simulink model "r2dbe_top"  (R2012b)
settings: Solver=VariableStepDiscrete  SolverMode=SingleTasking  StartTime=0.0  StopTime=10000  RelTol=1e-3
undefined symbols (not defined in the file or in its folder): r2dbe_vdif_lib, sfp, vdif
libraries: xbsIndex_r4 x2792, dspsigops x32, casper_library_delays x29, casper_library_sources x16, casper_library_misc x12, r2dbe_adc_lib x5, xps_library x4, simulink x2
(part 10 of 28)

== system r2dbe_top/r2dbe/tengbe_1/dest_ip ==
  sim_1 : Inport
  io_delay : xbsIndex_r4/Delay  rst=off  infoeditControl=Selection of Reset will increase slice count due to use of real FFs and instead of SRLs  en=off  latency=0  dbl_ovrd=off  reg_retiming=on  block_type=delay
  r2dbe_top_r2dbe_tengbe_1_dest_ip_user_data_out : xbsIndex_r4/Gateway In  gui_display_data_type=Fixed-point  arith_type=Unsigned  n_bits=32  bin_pt=0  preci_type=Single  exp_width=8  frac_width=24  quantization="Round  (unbiased: +/- Inf)"  overflow=Saturate  period=1  dbl_ovrd=off  timing_constraint=None  locs_specified=off  LOCs={}  UseAsADC=off  ADCChannel='1'  inherit_from_input=off  hdl_port=on  block_type=gatewayin
  reint1 : xbsIndex_r4/Reinterpret  force_arith_type=on  arith_type=Unsigned  force_bin_pt=on  bin_pt=0  block_type=reinterpret
  slice_ip : xbsIndex_r4/Slice  nbits=32  boolean_output=off  mode=Lower Bit Location + Width  bit1=0  base1=MSB of Input  bit0=0  base0=LSB of Input  dbl_ovrd=off  block_type=slice
  in_ip : Outport
  wires:
  r2dbe_top_r2dbe_tengbe_1_dest_ip_user_data_out/1 -> io_delay/1
  sim_1/1 -> r2dbe_top_r2dbe_tengbe_1_dest_ip_user_data_out/1
  io_delay/1 -> slice_ip/1
  slice_ip/1 -> reint1/1
  reint1/1 -> in_ip/1

== system r2dbe_top/r2dbe/tengbe_1/dest_port ==
  sim_1 : Inport
  io_delay : xbsIndex_r4/Delay  rst=off  infoeditControl=Selection of Reset will increase slice count due to use of real FFs and instead of SRLs  en=off  latency=0  dbl_ovrd=off  reg_retiming=on  block_type=delay
  r2dbe_top_r2dbe_tengbe_1_dest_port_user_data_out : xbsIndex_r4/Gateway In  gui_display_data_type=Fixed-point  arith_type=Unsigned  n_bits=32  bin_pt=0  preci_type=Single  exp_width=8  frac_width=24  quantization="Round  (unbiased: +/- Inf)"  overflow=Saturate  period=1  dbl_ovrd=off  timing_constraint=None  locs_specified=off  LOCs={}  UseAsADC=off  ADCChannel='1'  inherit_from_input=off  hdl_port=on  block_type=gatewayin
  reint1 : xbsIndex_r4/Reinterpret  force_arith_type=on  arith_type=Unsigned  force_bin_pt=on  bin_pt=0  block_type=reinterpret
  slice_port : xbsIndex_r4/Slice  nbits=16  boolean_output=off  mode=Lower Bit Location + Width  bit1=0  base1=MSB of Input  bit0=0  base0=LSB of Input  dbl_ovrd=off  block_type=slice
  in_port : Outport
  wires:
  r2dbe_top_r2dbe_tengbe_1_dest_port_user_data_out/1 -> io_delay/1
  sim_1/1 -> r2dbe_top_r2dbe_tengbe_1_dest_port_user_data_out/1
  io_delay/1 -> slice_port/1
  slice_port/1 -> reint1/1
  reint1/1 -> in_port/1

== system r2dbe_top/r2dbe/tengbe_1/rst ==
  sim_1 : Inport
  io_delay : xbsIndex_r4/Delay  rst=off  infoeditControl=Selection of Reset will increase slice count due to use of real FFs and instead of SRLs  en=off  latency=0  dbl_ovrd=off  reg_retiming=on  block_type=delay
  r2dbe_top_r2dbe_tengbe_1_rst_user_data_out : xbsIndex_r4/Gateway In  gui_display_data_type=Fixed-point  arith_type=Unsigned  n_bits=32  bin_pt=0  preci_type=Single  exp_width=8  frac_width=24  quantization="Round  (unbiased: +/- Inf)"  overflow=Saturate  period=1  dbl_ovrd=off  timing_constraint=None  locs_specified=off  LOCs={}  UseAsADC=off  ADCChannel='1'  inherit_from_input=off  hdl_port=on  block_type=gatewayin
  reint1 : xbsIndex_r4/Reinterpret  force_arith_type=on  arith_type=Unsigned  force_bin_pt=on  bin_pt=0  block_type=reinterpret
  slice_ip : xbsIndex_r4/Slice  nbits=32  boolean_output=off  mode=Lower Bit Location + Width  bit1=0  base1=MSB of Input  bit0=0  base0=LSB of Input  dbl_ovrd=off  block_type=slice
  in_ip : Outport
  wires:
  r2dbe_top_r2dbe_tengbe_1_rst_user_data_out/1 -> io_delay/1
  sim_1/1 -> r2dbe_top_r2dbe_tengbe_1_rst_user_data_out/1
  io_delay/1 -> slice_ip/1
  slice_ip/1 -> reint1/1
  reint1/1 -> in_ip/1

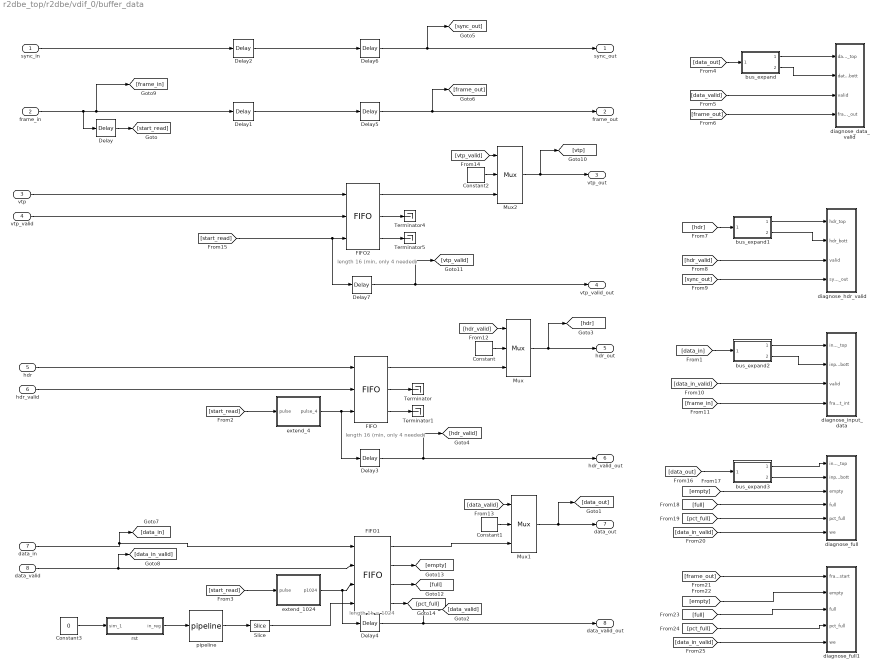
== system r2dbe_top/r2dbe/vdif_0/buffer_data ==
  note: length 1k = 1024
  note: length 16 (min, only 4 needed)
  note: length 16 (min, only 4 needed)
  sync_in : Inport
  frame_in : Inport  Port=2
  vtp : Inport  Port=3
  vtp_valid : Inport  Port=4
  hdr : Inport  Port=5
  hdr_valid : Inport  Port=6
  data_in : Inport  Port=7
  data_valid : Inport  Port=8
  Constant : xbsIndex_r4/Constant  const=0  gui_display_data_type=Fixed-point  arith_type=Unsigned  n_bits=64  bin_pt=0  preci_type=Single  exp_width=8  frac_width=24  explicit_period=on  period=1  equ=P=C  opselect=C  inp2=PCIN>>17  opr=+  inp1=P  carry=CIN  dbl_ovrd=off  block_type=constant
  Constant1 : xbsIndex_r4/Constant  const=0  gui_display_data_type=Fixed-point  arith_type=Unsigned  n_bits=64  bin_pt=0  preci_type=Single  exp_width=8  frac_width=24  explicit_period=on  period=1  equ=P=C  opselect=C  inp2=PCIN>>17  opr=+  inp1=P  carry=CIN  dbl_ovrd=off  block_type=constant
  Constant2 : xbsIndex_r4/Constant  const=0  gui_display_data_type=Fixed-point  arith_type=Unsigned  n_bits=64  bin_pt=0  preci_type=Single  exp_width=8  frac_width=24  explicit_period=on  period=1  equ=P=C  opselect=C  inp2=PCIN>>17  opr=+  inp1=P  carry=CIN  dbl_ovrd=off  block_type=constant
  Constant3 : Constant  Value=0
  Delay : xbsIndex_r4/Delay  rst=off  infoeditControl=Selection of Reset will increase slice count due to use of real FFs and instead of SRLs  en=off  latency=1024  dbl_ovrd=off  reg_retiming=off  block_type=delay
  Delay1 : xbsIndex_r4/Delay  rst=off  infoeditControl=Selection of Reset will increase slice count due to use of real FFs and instead of SRLs  en=off  latency=1024  dbl_ovrd=off  reg_retiming=off  block_type=delay
  Delay2 : xbsIndex_r4/Delay  rst=off  infoeditControl=Selection of Reset will increase slice count due to use of real FFs and instead of SRLs  en=off  latency=1024  dbl_ovrd=off  reg_retiming=off  block_type=delay
  Delay{3..7} (5 alike) : xbsIndex_r4/Delay  rst=off  infoeditControl=Selection of Reset will increase slice count due to use of real FFs and instead of SRLs  en=off  latency=1  dbl_ovrd=off  reg_retiming=off  block_type=delay
  FIFO : xbsIndex_r4/FIFO  mem_type=Block RAM  performance_options=Standard_FIFO  infoedit1=Available only for V4, V5, V6, V7, K7, A7 and Zynq devices.  embedded_registers=off  depth=16  percent_nbits=1  rst=off  en=off  use_dcount=off  use_percent_full_port=off  use_almost_empty=off  almost_empty_thresh=2  use_almost_full=off  almost_full_thresh=14  dbl_ovrd=off  explicit_period=off  block_type=fifo
  FIFO1 : xbsIndex_r4/FIFO  mem_type=Block RAM  performance_options=Standard_FIFO  infoedit1=Available only for V4, V5, V6, V7, K7, A7 and Zynq devices.  embedded_registers=off  depth=1K  percent_nbits=6  rst=on  en=off  use_dcount=off  use_percent_full_port=on  use_almost_empty=off  almost_empty_thresh=2  use_almost_full=off  almost_full_thresh=14  dbl_ovrd=off  explicit_period=off  block_type=fifo
  FIFO2 : xbsIndex_r4/FIFO  mem_type=Block RAM  performance_options=Standard_FIFO  infoedit1=Available only for V4, V5, V6, V7, K7, A7 and Zynq devices.  embedded_registers=off  depth=16  percent_nbits=1  rst=off  en=off  use_dcount=off  use_percent_full_port=off  use_almost_empty=off  almost_empty_thresh=2  use_almost_full=off  almost_full_thresh=14  dbl_ovrd=off  explicit_period=off  block_type=fifo
  Mux : xbsIndex_r4/Mux  inputs=2  en=off  latency=0  precision=Full  arith_type=Unsigned  n_bits=16  bin_pt=14  quantization=Truncate  overflow=Wrap  dbl_ovrd=off  block_type=mux
  Mux1 : xbsIndex_r4/Mux  inputs=2  en=off  latency=0  precision=Full  arith_type=Unsigned  n_bits=16  bin_pt=14  quantization=Truncate  overflow=Wrap  dbl_ovrd=off  block_type=mux
  Mux2 : xbsIndex_r4/Mux  inputs=2  en=off  latency=0  precision=Full  arith_type=Unsigned  n_bits=16  bin_pt=14  quantization=Truncate  overflow=Wrap  dbl_ovrd=off  block_type=mux
  Slice : xbsIndex_r4/Slice  nbits=1  boolean_output=on  mode=Lower Bit Location + Width  bit1=0  base1=LSB of Input  bit0=0  base0=LSB of Input  dbl_ovrd=off  block_type=slice
  Terminator{,1,4..5} (4 alike) : Terminator
  bus_expand : Subsystem  AncestorBlock=casper_library_flow_control/bus_expand  mask(bus_expand){mode=divisions of equal size, outputNum=2, outputWidth=32, outputBinaryPt=0, outputArithmeticType=0, show_format=off, outputToWorkspace=off, variablePrefix=out, outputToModelAsWell=on}
      mask prompts: outputNum "Number of outputs:"; outputWidth "Output width:"; outputBinaryPt "Output binary point position:"; outputArithmeticType "Output arithmetic type (ufix=0, fix=1, bool=2):"; show_format "Print format string?"; outputToWorkspace "Output to workspace?"; variablePrefix "Variable name prefix:"; outputToModelAsWell "Output to model as well?"
      mask help:
      | Expands a 'bus' made using a bus_create or Xilinx
      | concat block.
      | The input will be divided into the specified number
      | of outputs with the specified arithmetic types.
      | Divisions are made from most significant bit.
      mask init: same as r2dbe_top/r2dbe/delay_0/unbus
      settings: AttributesFormatString=2 outputs
      mask TypeOptions mode: divisions of equal size | divisions of arbitrary size
      mask Callback mode: bus_expand_callback();
      mask Callback outputWidth: bus_expand_callback();
      mask Callback outputToWorkspace: bus_expand_callback();
  bus_expand1 : Subsystem  AncestorBlock=casper_library_flow_control/bus_expand  mask(bus_expand){mode=divisions of equal size, outputNum=2, outputWidth=32, outputBinaryPt=0, outputArithmeticType=0, show_format=off, outputToWorkspace=off, variablePrefix=out, outputToModelAsWell=on}
      mask prompts: outputNum "Number of outputs:"; outputWidth "Output width:"; outputBinaryPt "Output binary point position:"; outputArithmeticType "Output arithmetic type (ufix=0, fix=1, bool=2):"; show_format "Print format string?"; outputToWorkspace "Output to workspace?"; variablePrefix "Variable name prefix:"; outputToModelAsWell "Output to model as well?"
      mask help:
      | Expands a 'bus' made using a bus_create or Xilinx
      | concat block.
      | The input will be divided into the specified number
      | of outputs with the specified arithmetic types.
      | Divisions are made from most significant bit.
      mask init: same as r2dbe_top/r2dbe/delay_0/unbus
      settings: AttributesFormatString=2 outputs
      mask TypeOptions mode: divisions of equal size | divisions of arbitrary size
      mask Callback mode: bus_expand_callback();
      mask Callback outputWidth: bus_expand_callback();
      mask Callback outputToWorkspace: bus_expand_callback();
  bus_expand2 : Subsystem  AncestorBlock=casper_library_flow_control/bus_expand  mask(bus_expand){mode=divisions of equal size, outputNum=2, outputWidth=32, outputBinaryPt=0, outputArithmeticType=0, show_format=off, outputToWorkspace=off, variablePrefix=out, outputToModelAsWell=on}
      mask prompts: outputNum "Number of outputs:"; outputWidth "Output width:"; outputBinaryPt "Output binary point position:"; outputArithmeticType "Output arithmetic type (ufix=0, fix=1, bool=2):"; show_format "Print format string?"; outputToWorkspace "Output to workspace?"; variablePrefix "Variable name prefix:"; outputToModelAsWell "Output to model as well?"
      mask help:
      | Expands a 'bus' made using a bus_create or Xilinx
      | concat block.
      | The input will be divided into the specified number
      | of outputs with the specified arithmetic types.
      | Divisions are made from most significant bit.
      mask init: same as r2dbe_top/r2dbe/delay_0/unbus
      settings: AttributesFormatString=2 outputs
      mask TypeOptions mode: divisions of equal size | divisions of arbitrary size
      mask Callback mode: bus_expand_callback();
      mask Callback outputWidth: bus_expand_callback();
      mask Callback outputToWorkspace: bus_expand_callback();
  bus_expand3 : Subsystem  AncestorBlock=casper_library_flow_control/bus_expand  mask(bus_expand){mode=divisions of equal size, outputNum=2, outputWidth=32, outputBinaryPt=0, outputArithmeticType=0, show_format=off, outputToWorkspace=off, variablePrefix=out, outputToModelAsWell=on}
      mask prompts: outputNum "Number of outputs:"; outputWidth "Output width:"; outputBinaryPt "Output binary point position:"; outputArithmeticType "Output arithmetic type (ufix=0, fix=1, bool=2):"; show_format "Print format string?"; outputToWorkspace "Output to workspace?"; variablePrefix "Variable name prefix:"; outputToModelAsWell "Output to model as well?"
      mask help:
      | Expands a 'bus' made using a bus_create or Xilinx
      | concat block.
      | The input will be divided into the specified number
      | of outputs with the specified arithmetic types.
      | Divisions are made from most significant bit.
      mask init: same as r2dbe_top/r2dbe/delay_0/unbus
      settings: AttributesFormatString=2 outputs
      mask TypeOptions mode: divisions of equal size | divisions of arbitrary size
      mask Callback mode: bus_expand_callback();
      mask Callback outputWidth: bus_expand_callback();
      mask Callback outputToWorkspace: bus_expand_callback();
  diagnose_data_valid : Subsystem
  diagnose_full : Subsystem
  diagnose_full1 : Subsystem
  diagnose_hdr_valid : Subsystem
  diagnose_input_data : Subsystem
  extend_1024 : Subsystem
  extend_4 : Subsystem
  pipeline : casper_library_delays/pipeline  latency=3
      settings: AttributesFormatString=Latency = %<latency>
  rst : Subsystem  Tag=xps:sw_reg  AncestorBlock=xps_library/software register  mask(swreg){mode=one value, io_dir=From Processor, io_delay=0, sample_period=1, names=reg, bitwidths=32, arith_types=0, bin_pts=0, sim_port=on, show_format=off}
      mask prompts: io_dir "I/O direction"; io_delay "I/O delay"; sample_period "Sample period"; names "Name:"; bitwidths "Bitwidth:"; arith_types "Type (ufix=0, fix=1, bool=2):"; bin_pts "Binary pt:"; sim_port "Provide sim input/output?"; show_format "Print format string?"
      mask init:
      | swreg_init(gcb)
      settings: AttributesFormatString=1input
      mask TypeOptions mode: one value | fields of equal size | fields of arbitrary size
      mask Callback mode: swreg_cb(gcb);
      mask TypeOptions io_dir: To Processor | From Processor
      mask Callback io_dir:
      | mask_enables = get_param(gcb, 'MaskEnables');
      | mask_names = get_param(gcb, 'MaskNames');
      | if strcmp(get_param(gcb, 'io_dir'), 'To Processor'),
      |     mask_enables{ismember(mask_names, 'sample_period')} = 'off';
      | else
      |     mask_enables{ismember(mask_names, 'sample_period')} = 'on';
      | end
      | set_param(gcb, 'MaskEnables', mask_enables);
      mask Callback bitwidths:
      | swreg_maskcheck(gcb);
      | % blk = gcb;
      | % mode = get_param(blk, 'mode');
      | % current_widths = eval(get_param(blk, 'bitwidths'));
      | % if (strcmp(mode, 'one value') || strcmp(mode, 'fields of equal size')) && (length(current_widths) > 1),
      | %     error('Only one width may be specified for this mode.');
      | % elseif strcmp(mode, 'fields of arbitrary size')
      | %     current_names = textscan(strtrim(strrep(strrep(get_param(blk, 'names'), ']', ''), '[', '')), '%s');
      | %     current_names = current_names{1};
      | %     numios = length(current_names);
      | %     if length(current_widths) ~= numios,
      | %         error('%d field names specified, but %d widths?', numios, length(current_widths));
      | %     end
      | % end
      | % total_width = 0;
      | % for ctr = 1 : length(current_widths),
      | %     total_width = total_width + current_widths(ctr);
      | % end
      | % if total_width > 32,
      | %     error('Total width must be 32 or less, set to %d.', total_width);
      | % end
      mask Callback arith_types:
      | [numios, ~, ~, ~, current_types] = swreg_maskcheck(gcb);
      | % blk = gcb;
      | % mode = get_param(blk, 'mode');
      | % current_types = eval(get_param(blk, 'arith_types'));
      | % numios = length(current_types);
      | % if (strcmp(mode, 'one value') || strcmp(mode, 'fields of equal size')) && (length(current_types) > 1),
      | %     error('Only one type may be specified for this mode.');
      | % elseif strcmp(mode, 'fields of arbitrary size')
      | %     current_names = textscan(strtrim(strrep(strrep(get_param(blk, 'names'), ']', ''), '[', '')), '%s');
      | %     current_names = current_names{1};
      | %     numios = length(current_names);
      | %     if length(current_types) ~= numios,
      | %         error('%d field names specified, but %d types?', numios, length(current_types));
      | %     end
      | % end
      | problem = 0;
      | for ctr = 1 : numios,
      |     t = current_types(ctr);
      |     if (t < 0) || (t > 2),
      |         problem = t;
      |         ctr = numios + 1;
      |     end
      | end
      | if problem ~= 0,
      |     error('Type cannot be %i, must be 0, 1 or 2.', problem);
      | end
      mask Callback bin_pts:
      | swreg_maskcheck(gcb);
      | % blk = gcb;
      | % mode = get_param(blk, 'mode');
      | % current_bins = eval(get_param(blk, 'bin_pts'));
      | % if (strcmp(mode, 'one value') || strcmp(mode, 'fields of equal size')) && (length(current_bins) > 1),
      | %     error('Only one binary pt may be specified for this mode.');
      | % elseif strcmp(mode, 'fields of arbitrary size')
      | %     current_names = textscan(strtrim(strrep(strrep(get_param(blk, 'names'), ']', ''), '[', '')), '%s');
      | %     current_names = current_names{1};
      | %     numios = length(current_names);
      | %     if length(current_bins) ~= numios,
      | %         error('%d field names specified, but %d binary pts?', numios, length(current_bins));
      | %     end
      | % end
  sync_out : Outport
  frame_out : Outport  Port=2
  vtp_out : Outport  Port=3
  vtp_valid_out : Outport  Port=4
  hdr_out : Outport  Port=5
  hdr_valid_out : Outport  Port=6
  data_out : Outport  Port=7
  data_valid_out : Outport  Port=8
  wires:
  sync_in/1 -> Delay2/1
  Delay/1 -> [start_read]
  hdr/1 -> FIFO/1
  hdr_valid/1 -> FIFO/2
  [start_read] -> extend_4/1(pulse)
  extend_4/1(pulse_4) -> Delay3/1, FIFO/3
  FIFO/1 -> Mux/3
  data_in/1 -> [data_in], FIFO1/1
  data_valid/1 -> [data_in_valid], FIFO1/2
  [start_read] -> extend_1024/1(pulse)
  extend_1024/1(p1024) -> Delay4/1, FIFO1/3
  FIFO1/1 -> Mux1/3
  FIFO/2 -> Terminator/1
  FIFO/3 -> Terminator1/1
  FIFO1/2 -> [empty]
  FIFO1/3 -> [full]
  bus_expand/2(lsb_out1) -> diagnose_data_valid/2(data_bott)
  bus_expand/1(msb_out2) -> diagnose_data_valid/1(data_top)
  [data_valid] -> diagnose_data_valid/3(valid)
  [frame_out] -> diagnose_data_valid/4(frame_start_out)
  [data_out] -> bus_expand/1(bus_in)
  frame_in/1 -> Delay/1, [frame_in], Delay1/1
  bus_expand1/2(lsb_out1) -> diagnose_hdr_valid/2(hdr_bott)
  bus_expand1/1(msb_out2) -> diagnose_hdr_valid/1(hdr_top)
  [hdr_valid] -> diagnose_hdr_valid/3(valid)
  [sync_out] -> diagnose_hdr_valid/4(sync_out)
  [hdr] -> bus_expand1/1(bus_in)
  Delay1/1 -> Delay5/1
  Delay2/1 -> Delay6/1
  bus_expand2/2(lsb_out1) -> diagnose_input_data/2(input_data_bott)
  bus_expand2/1(msb_out2) -> diagnose_input_data/1(input_data_top)
  [data_in_valid] -> diagnose_input_data/3(valid)
  [frame_in] -> diagnose_input_data/4(frame_start_int)
  [data_in] -> bus_expand2/1(bus_in)
  Delay3/1 -> hdr_valid_out/1, [hdr_valid]
  Delay4/1 -> data_valid_out/1, [data_valid]
  Delay5/1 -> frame_out/1, [frame_out]
  Delay6/1 -> [sync_out], sync_out/1
  Constant/1 -> Mux/2
  Mux/1 -> hdr_out/1, [hdr]
  [hdr_valid] -> Mux/1
  Constant1/1 -> Mux1/2
  [data_valid] -> Mux1/1
  Mux1/1 -> data_out/1, [data_out]
  vtp/1 -> FIFO2/1
  vtp_valid/1 -> FIFO2/2
  [start_read] -> FIFO2/3, Delay7/1
  FIFO2/1 -> Mux2/3
  FIFO2/2 -> Terminator4/1
  FIFO2/3 -> Terminator5/1
  Delay7/1 -> vtp_valid_out/1, [vtp_valid]
  Constant2/1 -> Mux2/2
  Mux2/1 -> vtp_out/1, [vtp]
  [vtp_valid] -> Mux2/1
  bus_expand3/2(lsb_out1) -> diagnose_full/2(input_data_bott)
  bus_expand3/1(msb_out2) -> diagnose_full/1(input_data_top)
  [empty] -> diagnose_full/3(empty)
  [full] -> diagnose_full/4(full)
  [data_out] -> bus_expand3/1(bus_in)
  [pct_full] -> diagnose_full/5(pct_full)
  [data_in_valid] -> diagnose_full/6(we)
  FIFO1/4 -> [pct_full]
  [empty] -> diagnose_full1/2(empty)
  [full] -> diagnose_full1/3(full)
  [pct_full] -> diagnose_full1/4(pct_full)
  [data_in_valid] -> diagnose_full1/5(we)
  [frame_out] -> diagnose_full1/1(frame_start)
  rst/1(in_reg) -> pipeline/1
  pipeline/1 -> Slice/1
  Constant3/1 -> rst/1(sim_1)
  Slice/1 -> FIFO1/4

== system r2dbe_top/r2dbe/vdif_0/delay_data ==
  sync_in : Inport
  frame_in : Inport  Port=2
  vtp : Inport  Port=3
  vtp_valid : Inport  Port=4
  hdr : Inport  Port=5
  hdr_valid : Inport  Port=6
  data : Inport  Port=7
  data_valid : Inport  Port=8
  Delay : xbsIndex_r4/Delay  rst=off  infoeditControl=Selection of Reset will increase slice count due to use of real FFs and instead of SRLs  en=off  latency=4  dbl_ovrd=off  reg_retiming=off  block_type=delay
  Delay1 : xbsIndex_r4/Delay  rst=off  infoeditControl=Selection of Reset will increase slice count due to use of real FFs and instead of SRLs  en=off  latency=4  dbl_ovrd=off  reg_retiming=off  block_type=delay
  Delay{2..5} (4 alike) : xbsIndex_r4/Delay  rst=off  infoeditControl=Selection of Reset will increase slice count due to use of real FFs and instead of SRLs  en=off  latency=1  dbl_ovrd=off  reg_retiming=off  block_type=delay
  bus_expand : Subsystem  AncestorBlock=casper_library_flow_control/bus_expand  mask(bus_expand){mode=divisions of equal size, outputNum=2, outputWidth=32, outputBinaryPt=0, outputArithmeticType=0, show_format=off, outputToWorkspace=off, variablePrefix=out, outputToModelAsWell=on}
      mask prompts: outputNum "Number of outputs:"; outputWidth "Output width:"; outputBinaryPt "Output binary point position:"; outputArithmeticType "Output arithmetic type (ufix=0, fix=1, bool=2):"; show_format "Print format string?"; outputToWorkspace "Output to workspace?"; variablePrefix "Variable name prefix:"; outputToModelAsWell "Output to model as well?"
      mask help:
      | Expands a 'bus' made using a bus_create or Xilinx
      | concat block.
      | The input will be divided into the specified number
      | of outputs with the specified arithmetic types.
      | Divisions are made from most significant bit.
      mask init: same as r2dbe_top/r2dbe/delay_0/unbus
      settings: AttributesFormatString=2 outputs
      mask TypeOptions mode: divisions of equal size | divisions of arbitrary size
      mask Callback mode: bus_expand_callback();
      mask Callback outputWidth: bus_expand_callback();
      mask Callback outputToWorkspace: bus_expand_callback();
  bus_expand1 : Subsystem  AncestorBlock=casper_library_flow_control/bus_expand  mask(bus_expand){mode=divisions of equal size, outputNum=2, outputWidth=32, outputBinaryPt=0, outputArithmeticType=0, show_format=off, outputToWorkspace=off, variablePrefix=out, outputToModelAsWell=on}
      mask prompts: outputNum "Number of outputs:"; outputWidth "Output width:"; outputBinaryPt "Output binary point position:"; outputArithmeticType "Output arithmetic type (ufix=0, fix=1, bool=2):"; show_format "Print format string?"; outputToWorkspace "Output to workspace?"; variablePrefix "Variable name prefix:"; outputToModelAsWell "Output to model as well?"
      mask help:
      | Expands a 'bus' made using a bus_create or Xilinx
      | concat block.
      | The input will be divided into the specified number
      | of outputs with the specified arithmetic types.
      | Divisions are made from most significant bit.
      mask init: same as r2dbe_top/r2dbe/delay_0/unbus
      settings: AttributesFormatString=2 outputs
      mask TypeOptions mode: divisions of equal size | divisions of arbitrary size
      mask Callback mode: bus_expand_callback();
      mask Callback outputWidth: bus_expand_callback();
      mask Callback outputToWorkspace: bus_expand_callback();
  diagnose_data_valid : Subsystem
  diagnose_data_valid1 : Subsystem
  sync_out : Outport
  frame_out : Outport  Port=2
  vtp_out : Outport  Port=3
  vtp_valid_out : Outport  Port=4
  hdr_out : Outport  Port=5
  hdr_out_valid : Outport  Port=6
  data_out : Outport  Port=7
  data_out_valid : Outport  Port=8
  wires:
  [data_out] -> bus_expand/1(bus_in)
  bus_expand/1(msb_out2) -> diagnose_data_valid/1(data_top)
  bus_expand/2(lsb_out1) -> diagnose_data_valid/2(data_bott)
  sync_in/1 -> [sync_out], sync_out/1
  frame_in/1 -> [frame_out], frame_out/1
  hdr/1 -> Delay3/1
  hdr_valid/1 -> Delay2/1
  data/1 -> Delay4/1
  Delay/1 -> [data_out], data_out/1
  data_valid/1 -> Delay5/1
  Delay1/1 -> [data_valid], data_out_valid/1
  [hdr] -> bus_expand1/1(bus_in)
  bus_expand1/1(msb_out2) -> diagnose_data_valid/4(hdr_top)
  bus_expand1/2(lsb_out1) -> diagnose_data_valid/5(hdr_bott)
  [data_valid] -> diagnose_data_valid/3(data_valid)
  [hdr_valid] -> diagnose_data_valid/6(hdr_valid)
  [sync_out] -> diagnose_data_valid1/1(sync)
  [frame_out] -> diagnose_data_valid1/2(frame)
  [data_valid] -> diagnose_data_valid1/3(data_valid)
  [hdr_valid] -> diagnose_data_valid1/4(hdr_valid)
  vtp/1 -> vtp_out/1, [vtp]
  vtp_valid/1 -> vtp_valid_out/1, [vtp_valid]
  Delay2/1 -> [hdr_valid], hdr_out_valid/1
  Delay3/1 -> [hdr], hdr_out/1
  Delay4/1 -> Delay/1
  Delay5/1 -> Delay1/1

== system r2dbe_top/r2dbe/vdif_0/enable ==
  sim_1 : Inport
  io_delay : xbsIndex_r4/Delay  rst=off  infoeditControl=Selection of Reset will increase slice count due to use of real FFs and instead of SRLs  en=off  latency=0  dbl_ovrd=off  reg_retiming=on  block_type=delay
  r2dbe_top_r2dbe_vdif_0_enable_user_data_out : xbsIndex_r4/Gateway In  gui_display_data_type=Fixed-point  arith_type=Unsigned  n_bits=32  bin_pt=0  preci_type=Single  exp_width=8  frac_width=24  quantization="Round  (unbiased: +/- Inf)"  overflow=Saturate  period=1  dbl_ovrd=off  timing_constraint=None  locs_specified=off  LOCs={}  UseAsADC=off  ADCChannel='1'  inherit_from_input=off  hdl_port=on  block_type=gatewayin
  reint1 : xbsIndex_r4/Reinterpret  force_arith_type=on  arith_type=Unsigned  force_bin_pt=on  bin_pt=0  block_type=reinterpret
  slice_reg : xbsIndex_r4/Slice  nbits=32  boolean_output=off  mode=Lower Bit Location + Width  bit1=0  base1=MSB of Input  bit0=0  base0=LSB of Input  dbl_ovrd=off  block_type=slice
  in_reg : Outport
  wires:
  r2dbe_top_r2dbe_vdif_0_enable_user_data_out/1 -> io_delay/1
  sim_1/1 -> r2dbe_top_r2dbe_vdif_0_enable_user_data_out/1
  io_delay/1 -> slice_reg/1
  slice_reg/1 -> reint1/1
  reint1/1 -> in_reg/1

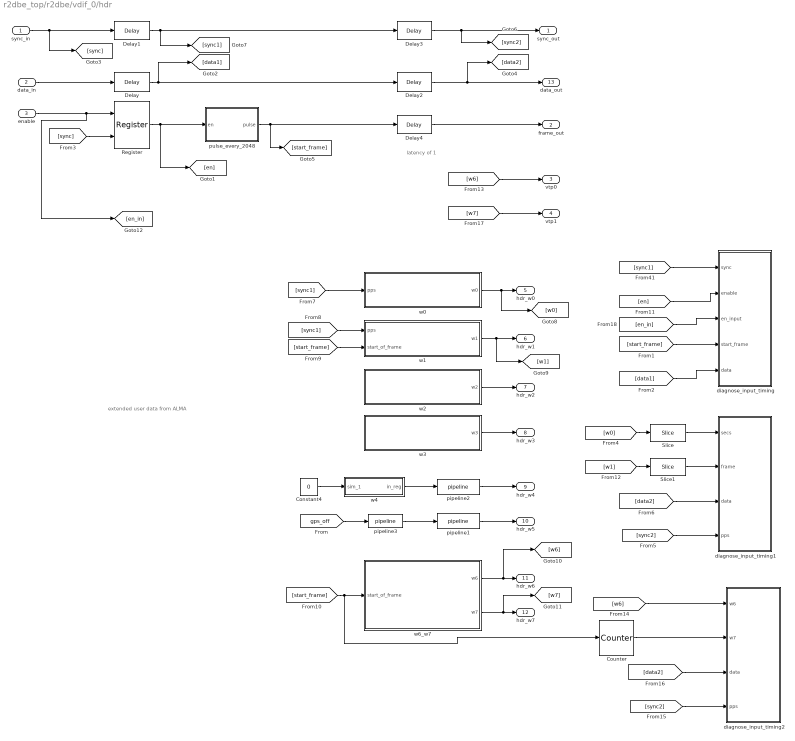
== system r2dbe_top/r2dbe/vdif_0/hdr ==
  note: latency of 1
  note: extended user data
      | from ALMA
  sync_in : Inport
  data_in : Inport  Port=2
  enable : Inport  Port=3
  Constant4 : Constant  Value=0
  Counter : xbsIndex_r4/Counter  cnt_type=Free Running  cnt_to=Inf  operation=Up  start_count=2^32-1  cnt_by_val=1  arith_type=Unsigned  n_bits=32  bin_pt=0  load_pin=off  rst=off  en=on  explicit_period=on  period=1  dbl_ovrd=off  use_behavioral_HDL=off  implementation=Fabric  block_type=counter
  Delay{,1..4} (5 alike) : xbsIndex_r4/Delay  rst=off  infoeditControl=Selection of Reset will increase slice count due to use of real FFs and instead of SRLs  en=off  latency=1  dbl_ovrd=off  reg_retiming=off  block_type=delay
  Register : xbsIndex_r4/Register  init=0  rst=off  en=on  dbl_ovrd=off  block_type=register
  Slice : xbsIndex_r4/Slice  nbits=30  boolean_output=off  mode=Lower Bit Location + Width  bit1=0  base1=MSB of Input  bit0=0  base0=LSB of Input  dbl_ovrd=off  block_type=slice
  Slice1 : xbsIndex_r4/Slice  nbits=24  boolean_output=off  mode=Lower Bit Location + Width  bit1=0  base1=MSB of Input  bit0=0  base0=LSB of Input  dbl_ovrd=off  block_type=slice
  diagnose_input_timing : Subsystem
  diagnose_input_timing1 : Subsystem
  diagnose_input_timing2 : Subsystem
  pipeline1 : casper_library_delays/pipeline  latency=1
      settings: AttributesFormatString=Latency = %<latency>
  pipeline2 : casper_library_delays/pipeline  latency=1
      settings: AttributesFormatString=Latency = %<latency>
  pipeline3 : casper_library_delays/pipeline  latency=3
      settings: AttributesFormatString=Latency = %<latency>
  pulse_every_2048 : Subsystem  mask{per=2048}
      mask prompts: per "period"
      mask help: Creates a pulse duration 1 with period from 2 to <large number>. Pulse begins with enable signal, no latency.
  w0 : Subsystem
  w1 : Subsystem
  w2 : Subsystem
  w3 : Subsystem
  w4 : Subsystem  Tag=xps:sw_reg  AncestorBlock=xps_library/software register  mask(swreg){mode=one value, io_dir=From Processor, io_delay=0, sample_period=1, names=reg, bitwidths=32, arith_types=0, bin_pts=0, sim_port=on, show_format=off}
      mask prompts: io_dir "I/O direction"; io_delay "I/O delay"; sample_period "Sample period"; names "Name:"; bitwidths "Bitwidth:"; arith_types "Type (ufix=0, fix=1, bool=2):"; bin_pts "Binary pt:"; sim_port "Provide sim input/output?"; show_format "Print format string?"
      mask init:
      | swreg_init(gcb)
      settings: AttributesFormatString=1input
      mask TypeOptions mode: one value | fields of equal size | fields of arbitrary size
      mask Callback mode: swreg_cb(gcb);
      mask TypeOptions io_dir: To Processor | From Processor
      mask Callback io_dir:
      | mask_enables = get_param(gcb, 'MaskEnables');
      | mask_names = get_param(gcb, 'MaskNames');
      | if strcmp(get_param(gcb, 'io_dir'), 'To Processor'),
      |     mask_enables{ismember(mask_names, 'sample_period')} = 'off';
      | else
      |     mask_enables{ismember(mask_names, 'sample_period')} = 'on';
      | end
      | set_param(gcb, 'MaskEnables', mask_enables);
      mask Callback bitwidths:
      | swreg_maskcheck(gcb);
      | % blk = gcb;
      | % mode = get_param(blk, 'mode');
      | % current_widths = eval(get_param(blk, 'bitwidths'));
      | % if (strcmp(mode, 'one value') || strcmp(mode, 'fields of equal size')) && (length(current_widths) > 1),
      | %     error('Only one width may be specified for this mode.');
      | % elseif strcmp(mode, 'fields of arbitrary size')
      | %     current_names = textscan(strtrim(strrep(strrep(get_param(blk, 'names'), ']', ''), '[', '')), '%s');
      | %     current_names = current_names{1};
      | %     numios = length(current_names);
      | %     if length(current_widths) ~= numios,
      | %         error('%d field names specified, but %d widths?', numios, length(current_widths));
      | %     end
      | % end
      | % total_width = 0;
      | % for ctr = 1 : length(current_widths),
      | %     total_width = total_width + current_widths(ctr);
      | % end
      | % if total_width > 32,
      | %     error('Total width must be 32 or less, set to %d.', total_width);
      | % end
      mask Callback arith_types:
      | [numios, ~, ~, ~, current_types] = swreg_maskcheck(gcb);
      | % blk = gcb;
      | % mode = get_param(blk, 'mode');
      | % current_types = eval(get_param(blk, 'arith_types'));
      | % numios = length(current_types);
      | % if (strcmp(mode, 'one value') || strcmp(mode, 'fields of equal size')) && (length(current_types) > 1),
      | %     error('Only one type may be specified for this mode.');
      | % elseif strcmp(mode, 'fields of arbitrary size')
      | %     current_names = textscan(strtrim(strrep(strrep(get_param(blk, 'names'), ']', ''), '[', '')), '%s');
      | %     current_names = current_names{1};
      | %     numios = length(current_names);
      | %     if length(current_types) ~= numios,
      | %         error('%d field names specified, but %d types?', numios, length(current_types));
      | %     end
      | % end
      | problem = 0;
      | for ctr = 1 : numios,
      |     t = current_types(ctr);
      |     if (t < 0) || (t > 2),
      |         problem = t;
      |         ctr = numios + 1;
      |     end
      | end
      | if problem ~= 0,
      |     error('Type cannot be %i, must be 0, 1 or 2.', problem);
      | end
      mask Callback bin_pts:
      | swreg_maskcheck(gcb);
      | % blk = gcb;
      | % mode = get_param(blk, 'mode');
      | % current_bins = eval(get_param(blk, 'bin_pts'));
      | % if (strcmp(mode, 'one value') || strcmp(mode, 'fields of equal size')) && (length(current_bins) > 1),
      | %     error('Only one binary pt may be specified for this mode.');
      | % elseif strcmp(mode, 'fields of arbitrary size')
      | %     current_names = textscan(strtrim(strrep(strrep(get_param(blk, 'names'), ']', ''), '[', '')), '%s');
      | %     current_names = current_names{1};
      | %     numios = length(current_names);
      | %     if length(current_bins) ~= numios,
      | %         error('%d field names specified, but %d binary pts?', numios, length(current_bins));
      | %     end
      | % end
  w6_w7 : Subsystem
  sync_out : Outport
  frame_out : Outport  Port=2
  vtp0 : Outport  Port=3
  vtp1 : Outport  Port=4
  hdr_w0 : Outport  Port=5
  hdr_w1 : Outport  Port=6
  hdr_w2 : Outport  Port=7
  hdr_w3 : Outport  Port=8
  hdr_w4 : Outport  Port=9
  hdr_w5 : Outport  Port=10
  hdr_w6 : Outport  Port=11
  hdr_w7 : Outport  Port=12
  data_out : Outport  Port=13
  wires:
  [gps_off] -> pipeline3/1
  w4/1(in_reg) -> pipeline2/1
  Constant4/1 -> w4/1(sim_1)
  [en] -> diagnose_input_timing/2(enable)
  [sync1] -> diagnose_input_timing/1(sync)
  [start_frame] -> w1/2(start_of_frame)
  [sync1] -> w1/1(pps)
  [sync1] -> w0/1(pps)
  sync_in/1 -> [sync], Delay1/1
  data_in/1 -> Delay/1
  w0/1(w0) -> hdr_w0/1, [w0]
  w1/1(w1) -> hdr_w1/1, [w1]
  w2/1(w2) -> hdr_w2/1
  w3/1(w3) -> hdr_w3/1
  pipeline2/1 -> hdr_w4/1
  pipeline1/1 -> hdr_w5/1
  w6_w7/1(w6) -> hdr_w6/1, [w6]
  w6_w7/2(w7) -> hdr_w7/1, [w7]
  [start_frame] -> Counter/1, w6_w7/1(start_of_frame)
  pulse_every_2048/1(pulse) -> Delay4/1, [start_frame]
  enable/1 -> [en_in], Register/1
  [sync] -> Register/2
  Register/1 -> [en], pulse_every_2048/1(en)
  Delay/1 -> [data1], Delay2/1
  Delay1/1 -> Delay3/1, [sync1]
  Slice1/1 -> diagnose_input_timing1/2(frame)
  Slice/1 -> diagnose_input_timing1/1(secs)
  [data2] -> diagnose_input_timing1/3(data)
  [sync2] -> diagnose_input_timing1/4(pps)
  Delay2/1 -> data_out/1, [data2]
  Delay3/1 -> [sync2], sync_out/1
  [w0] -> Slice/1
  [w1] -> Slice1/1
  Delay4/1 -> frame_out/1
  Counter/1 -> diagnose_input_timing2/2(w7)
  [w6] -> diagnose_input_timing2/1(w6)
  [data2] -> diagnose_input_timing2/3(data)
  [sync2] -> diagnose_input_timing2/4(pps)
  [w6] -> vtp0/1
  [w7] -> vtp1/1
  [en_in] -> diagnose_input_timing/3(en_input)
  [start_frame] -> diagnose_input_timing/4(start_frame)
  [data1] -> diagnose_input_timing/5(data)
  pipeline3/1 -> pipeline1/1

== system r2dbe_top/r2dbe/vdif_0/little_end ==
  sim_1 : Inport
  io_delay : xbsIndex_r4/Delay  rst=off  infoeditControl=Selection of Reset will increase slice count due to use of real FFs and instead of SRLs  en=off  latency=0  dbl_ovrd=off  reg_retiming=on  block_type=delay
  r2dbe_top_r2dbe_vdif_0_little_end_user_data_out : xbsIndex_r4/Gateway In  gui_display_data_type=Fixed-point  arith_type=Unsigned  n_bits=32  bin_pt=0  preci_type=Single  exp_width=8  frac_width=24  quantization="Round  (unbiased: +/- Inf)"  overflow=Saturate  period=1  dbl_ovrd=off  timing_constraint=None  locs_specified=off  LOCs={}  UseAsADC=off  ADCChannel='1'  inherit_from_input=off  hdl_port=on  block_type=gatewayin
  reint1 : xbsIndex_r4/Reinterpret  force_arith_type=on  arith_type=Unsigned  force_bin_pt=on  bin_pt=0  block_type=reinterpret
  slice_reg : xbsIndex_r4/Slice  nbits=32  boolean_output=off  mode=Lower Bit Location + Width  bit1=0  base1=MSB of Input  bit0=0  base0=LSB of Input  dbl_ovrd=off  block_type=slice
  in_reg : Outport
  wires:
  r2dbe_top_r2dbe_vdif_0_little_end_user_data_out/1 -> io_delay/1
  sim_1/1 -> r2dbe_top_r2dbe_vdif_0_little_end_user_data_out/1
  io_delay/1 -> slice_reg/1
  slice_reg/1 -> reint1/1
  reint1/1 -> in_reg/1

== system r2dbe_top/r2dbe/vdif_0/mk_64_from_32 ==
  sync_in : Inport
  frame_start : Inport  Port=2
  vtp : Inport  Port=3
  vtp_valid : Inport  Port=4
  hdr : Inport  Port=5
  hdr_valid : Inport  Port=6
  data_in : Inport  Port=7
  data_valid : Inport  Port=8
  Delay{,1..4} (5 alike) : xbsIndex_r4/Delay  rst=off  infoeditControl=Selection of Reset will increase slice count due to use of real FFs and instead of SRLs  en=off  latency=2  dbl_ovrd=off  reg_retiming=off  block_type=delay
  Logical : xbsIndex_r4/Logical  logical_function=AND  inputs=2  en=off  latency=0  precision=Full  arith_type=Unsigned  n_bits=16  bin_pt=0  align_bp=on  dbl_ovrd=off  block_type=logical
  Logical1 : xbsIndex_r4/Logical  logical_function=AND  inputs=2  en=off  latency=0  precision=Full  arith_type=Unsigned  n_bits=16  bin_pt=0  align_bp=on  dbl_ovrd=off  block_type=logical
  Logical2 : xbsIndex_r4/Logical  logical_function=AND  inputs=2  en=off  latency=0  precision=Full  arith_type=Unsigned  n_bits=16  bin_pt=0  align_bp=on  dbl_ovrd=off  block_type=logical
  bus_expand : Subsystem  AncestorBlock=casper_library_flow_control/bus_expand  mask(bus_expand){mode=divisions of equal size, outputNum=2, outputWidth=32, outputBinaryPt=0, outputArithmeticType=0, show_format=off, outputToWorkspace=off, variablePrefix=out, outputToModelAsWell=on}
      mask prompts: outputNum "Number of outputs:"; outputWidth "Output width:"; outputBinaryPt "Output binary point position:"; outputArithmeticType "Output arithmetic type (ufix=0, fix=1, bool=2):"; show_format "Print format string?"; outputToWorkspace "Output to workspace?"; variablePrefix "Variable name prefix:"; outputToModelAsWell "Output to model as well?"
      mask help:
      | Expands a 'bus' made using a bus_create or Xilinx
      | concat block.
      | The input will be divided into the specified number
      | of outputs with the specified arithmetic types.
      | Divisions are made from most significant bit.
      mask init: same as r2dbe_top/r2dbe/delay_0/unbus
      settings: AttributesFormatString=2 outputs
      mask TypeOptions mode: divisions of equal size | divisions of arbitrary size
      mask Callback mode: bus_expand_callback();
      mask Callback outputWidth: bus_expand_callback();
      mask Callback outputToWorkspace: bus_expand_callback();
  bus_expand1 : Subsystem  AncestorBlock=casper_library_flow_control/bus_expand  mask(bus_expand){mode=divisions of equal size, outputNum=2, outputWidth=32, outputBinaryPt=0, outputArithmeticType=0, show_format=off, outputToWorkspace=off, variablePrefix=out, outputToModelAsWell=on}
      mask prompts: outputNum "Number of outputs:"; outputWidth "Output width:"; outputBinaryPt "Output binary point position:"; outputArithmeticType "Output arithmetic type (ufix=0, fix=1, bool=2):"; show_format "Print format string?"; outputToWorkspace "Output to workspace?"; variablePrefix "Variable name prefix:"; outputToModelAsWell "Output to model as well?"
      mask help:
      | Expands a 'bus' made using a bus_create or Xilinx
      | concat block.
      | The input will be divided into the specified number
      | of outputs with the specified arithmetic types.
      | Divisions are made from most significant bit.
      mask init: same as r2dbe_top/r2dbe/delay_0/unbus
      settings: AttributesFormatString=2 outputs
      mask TypeOptions mode: divisions of equal size | divisions of arbitrary size
      mask Callback mode: bus_expand_callback();
      mask Callback outputWidth: bus_expand_callback();
      mask Callback outputToWorkspace: bus_expand_callback();
  diagnose_data_valid : Subsystem
  diagnose_hdr_valid : Subsystem
  stack_1 : Subsystem
      mask help: stacks 2 samples together, based on a flag that indicates the start or the first sample of data to be stacked. outputs the stacked data and a valid signal, such that on any given valid signal the data represents the newest data in the top half and the oldest data in the lower half. Therefore given a data stream starting with 0, increasing by 1 every clock cycle I would expect the first data valid to indicate a piece of data with the value 0 in the low bits, 1 in the high, and the next sample having 2 in the low bits 3 in the high, etc.
  stack_2 : Subsystem
      mask help: stacks 2 samples together, based on a flag that indicates the start or the first sample of data to be stacked. outputs the stacked data and a valid signal, such that on any given valid signal the data represents the newest data in the top half and the oldest data in the lower half. Therefore given a data stream starting with 0, increasing by 1 every clock cycle I would expect the first data valid to indicate a piece of data with the value 0 in the low bits, 1 in the high, and the next sample having 2 in the low bits 3 in the high, etc.
  stack_3 : Subsystem
      mask help: stacks 2 samples together, based on a flag that indicates the start or the first sample of data to be stacked. outputs the stacked data and a valid signal, such that on any given valid signal the data represents the newest data in the top half and the oldest data in the lower half. Therefore given a data stream starting with 0, increasing by 1 every clock cycle I would expect the first data valid to indicate a piece of data with the value 0 in the low bits, 1 in the high, and the next sample having 2 in the low bits 3 in the high, etc.
  sync_out : Outport
  frame_out : Outport  Port=2
  vpt_out : Outport  Port=3
  vtp_valid_out : Outport  Port=4
  hdr_out : Outport  Port=5
  hdr_valid_out : Outport  Port=6
  data_out : Outport  Port=7
  data_valid_out : Outport  Port=8
  wires:
  data_in/1 -> stack_2/1(value)
  frame_start/1 -> [start], Delay/1
  [start] -> stack_2/2(start)
  sync_in/1 -> Delay2/1
  stack_2/1(value_2) -> data_out/1, [data_out]
  [start] -> stack_1/2(start)
  stack_1/1(value_2) -> hdr_out/1, [hdr]
  stack_1/2(valid) -> Logical/1
  Delay/1 -> [frame_out], frame_out/1
  bus_expand/2(lsb_out1) -> diagnose_data_valid/2(data_bott)
  bus_expand/1(msb_out2) -> diagnose_data_valid/1(data_top)
  [data_valid] -> diagnose_data_valid/3(valid)
  [frame_out] -> diagnose_data_valid/4(frame_start_out)
  [data_out] -> bus_expand/1(bus_in)
  bus_expand1/2(lsb_out1) -> diagnose_hdr_valid/2(data_bott)
  bus_expand1/1(msb_out2) -> diagnose_hdr_valid/1(data_top)
  [hdr_valid] -> diagnose_hdr_valid/3(valid)
  [sync_out] -> diagnose_hdr_valid/4(sync_out)
  [hdr] -> bus_expand1/1(bus_in)
  Logical/1 -> hdr_valid_out/1, [hdr_valid]
  Delay1/1 -> Logical/2
  Delay2/1 -> [sync_out], sync_out/1
  [start] -> stack_3/2(start)
  stack_3/1(value_2) -> vpt_out/1, [vtp]
  stack_3/2(valid) -> Logical1/1
  Logical1/1 -> vtp_valid_out/1, [vtp_valid]
  Delay3/1 -> Logical1/2
  vtp/1 -> stack_3/1(value)
  vtp_valid/1 -> Delay3/1
  hdr/1 -> stack_1/1(value)
  hdr_valid/1 -> Delay1/1
  data_valid/1 -> Delay4/1
  Delay4/1 -> Logical2/2
  stack_2/2(valid) -> Logical2/1
  Logical2/1 -> data_valid_out/1, [data_valid]

== system r2dbe_top/r2dbe/vdif_0/mk_tengbe_sigs ==
  note: logical OR the valid signals so that the
      | tx_valid is held high for 1024+4 = 1028 clocks
  note: delay to align with
      | negedge
  sync : Inport
  frame_start : Inport  Port=2
  vtp : Inport  Port=3
  vtp_valid : Inport  Port=4
  hdr : Inport  Port=5
  hdr_valid : Inport  Port=6
  data : Inport  Port=7
  data_valid : Inport  Port=8
  le : Inport  Port=9
  Delay{,1..3} (4 alike) : xbsIndex_r4/Delay  rst=off  infoeditControl=Selection of Reset will increase slice count due to use of real FFs and instead of SRLs  en=off  latency=1  dbl_ovrd=off  reg_retiming=off  block_type=delay
  Logical : xbsIndex_r4/Logical  logical_function=XOR  inputs=3  en=off  latency=0  precision=Full  arith_type=Unsigned  n_bits=16  bin_pt=0  align_bp=on  dbl_ovrd=off  block_type=logical
  Logical1 : xbsIndex_r4/Logical  logical_function=XOR  inputs=3  en=off  latency=0  precision=Full  arith_type=Unsigned  n_bits=16  bin_pt=0  align_bp=on  dbl_ovrd=off  block_type=logical
  Terminator : Terminator
  Terminator1 : Terminator
  bus_expand : Subsystem  AncestorBlock=casper_library_flow_control/bus_expand  mask(bus_expand){mode=divisions of equal size, outputNum=2, outputWidth=32, outputBinaryPt=0, outputArithmeticType=0, show_format=off, outputToWorkspace=off, variablePrefix=out, outputToModelAsWell=on}
      mask prompts: outputNum "Number of outputs:"; outputWidth "Output width:"; outputBinaryPt "Output binary point position:"; outputArithmeticType "Output arithmetic type (ufix=0, fix=1, bool=2):"; show_format "Print format string?"; outputToWorkspace "Output to workspace?"; variablePrefix "Variable name prefix:"; outputToModelAsWell "Output to model as well?"
      mask help:
      | Expands a 'bus' made using a bus_create or Xilinx
      | concat block.
      | The input will be divided into the specified number
      | of outputs with the specified arithmetic types.
      | Divisions are made from most significant bit.
      mask init: same as r2dbe_top/r2dbe/delay_0/unbus
      settings: AttributesFormatString=2 outputs
      mask TypeOptions mode: divisions of equal size | divisions of arbitrary size
      mask Callback mode: bus_expand_callback();
      mask Callback outputWidth: bus_expand_callback();
      mask Callback outputToWorkspace: bus_expand_callback();
  change_endianness : Subsystem
  diagnose_data_valid : Subsystem
  edge_detect : Subsystem  AncestorBlock=casper_library_misc/edge_detect  mask(edge_detect){edge=Falling, polarity=Active High, x_in=[0 0.08 0.08 0.16 0.16 0.24 0.24 0.32 0.32 0.4], y_in=[-1 -1  1  1  1  1  1  1  1  1], x_out=[0.6 0.68 0.68 0.76 0.76 0.84 0.84 0.92 0.92 1], y_out=[-1 -1  1  1 -1 -1 -1 -1 -1 -1]}
      mask prompts: edge "Edge Type"; polarity "Output Polarity"; x_in "Input X Positions"; y_in "Input Y Positions"; x_out "Output X Positions"; y_out "Output Y Positions"
      mask help: Output is active for one-cycle after each edge of the specified type (i.e. rising, falling or both).
      mask init:
      | edge_detect_init(gcb,...
      |     'edge',edge,...
      |     'polarity',polarity,...
      |     'x_in',x_in,...
      |     'x_out',x_out,...
      |     'y_in',y_in,...
      |     'y_out',y_out);
      | 
      | x_in_num=str2num(getfield(getfield(get_param(gcb,'UserData'),'parameters'),'x_in'));
      | x_out_num=str2num(getfield(getfield(get_param(gcb,'UserData'),'parameters'),'x_out'));
      | y_in_num=str2num(getfield(getfield(get_param(gcb,'UserData'),'parameters'),'y_in'));
      | y_out_num=str2num(getfield(getfield(get_param(gcb,'UserData'),'parameters'),'y_out'));
      settings: AttributesFormatString=|
      | falling edges
      | active high
      mask Help: Output is active for one-cycle after each edge of the specified type (i.e. rising, falling, or both).  Latency is zero.
      mask TypeOptions edge: Rising | Falling | Both
      mask TypeOptions polarity: Active High | Active Low
      mask Display:
      | plot(x_in_num,0.5+y_in_num*0.2);
      | plot(x_out_num,0.5+y_out_num*0.2);
  tx_data : Outport
  tx_valid : Outport  Port=2
  tx_eof : Outport  Port=3
  wires:
  edge_detect/1(out) -> tx_eof/1
  Logical1/1 -> edge_detect/1(in), Delay/1
  Delay/1 -> [data_valid], tx_valid/1
  Logical/1 -> change_endianness/1(be)
  change_endianness/1(data_out) -> Delay1/1
  [le] -> change_endianness/2(little_end)
  Delay2/1 -> Terminator1/1
  sync/1 -> Delay2/1
  Delay1/1 -> [data_out], tx_data/1
  frame_start/1 -> Delay3/1
  Delay3/1 -> [frame_out], Terminator/1
  bus_expand/2(lsb_out1) -> diagnose_data_valid/2(data_bott)
  bus_expand/1(msb_out2) -> diagnose_data_valid/1(data_top)
  [data_valid] -> diagnose_data_valid/3(valid)
  [frame_out] -> diagnose_data_valid/4(frame_start_out)
  [data_out] -> bus_expand/1(bus_in)
  hdr/1 -> Logical/2
  vtp/1 -> Logical/1
  data/1 -> Logical/3
  le/1 -> [le]
  vtp_valid/1 -> Logical1/1
  hdr_valid/1 -> Logical1/2
  data_valid/1 -> Logical1/3

== system r2dbe_top/r2dbe/vdif_0/reorder ==
  d_native : Inport
  Concat : xbsIndex_r4/Concat  num_inputs=16  dbl_ovrd=off  block_type=concat
  Subsystem : Subsystem
  d_ordered : Outport
  wires:
  Concat/1 -> d_ordered/1
  d_native/1 -> Subsystem/1(bus_in)
  Subsystem/1(msb_out16) -> Concat/16
  Subsystem/2(out15) -> Concat/15
  Subsystem/3(out14) -> Concat/14
  Subsystem/4(out13) -> Concat/13
  Subsystem/5(out12) -> Concat/12
  Subsystem/6(out11) -> Concat/11
  Subsystem/7(out10) -> Concat/10
  Subsystem/8(out9) -> Concat/9
  Subsystem/9(out8) -> Concat/8
  Subsystem/10(out7) -> Concat/7
  Subsystem/11(out6) -> Concat/6
  Subsystem/12(out5) -> Concat/5
  Subsystem/13(out4) -> Concat/4
  Subsystem/14(out3) -> Concat/3
  Subsystem/15(out2) -> Concat/2
  Subsystem/16(lsb_out1) -> Concat/1
